simulink model "test_loopback_buf"  (Simulink 6.2)
settings: Solver=ode45  StartTime=0.0  StopTime=4000  RelTol=1e-3
undefined symbols (not defined in the file): Down, Up
libraries: xbsIndex_r3 x1383, xps_library x52, casper_library x37
(part 6 of 8)

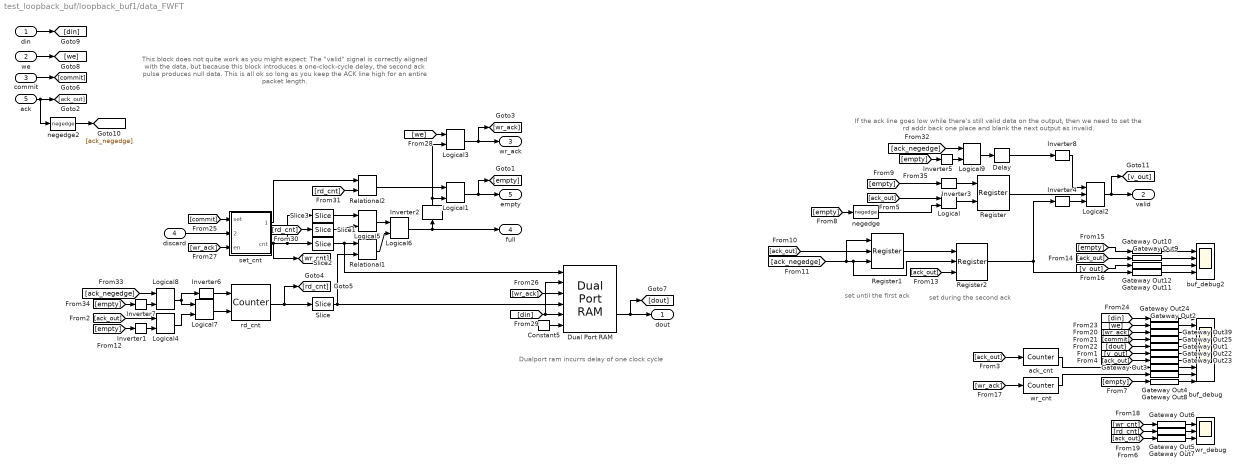
== system test_loopback_buf/loopback_buf1/data_FWFT ==
  note: This block does not quite work as you might expect:
      | The "valid" signal is correctly aligned with the data,
      | but because this block introduces a one-clock-cycle delay,
      | the second ack pulse produces null data.
      |
      | This is all ok so long as you keep the ACK line high for an entire packet length.
  note: set until the first ack
  note: set during the second ack
  note: If the ack line goes low while there's still valid data on the output,
      | then we need to set the rd addr back one place and blank the next
      | output as invalid.
  note: Dualport ram incurrs delay
      | of one clock cycle
  din : Inport  Port=1  LatchInput=off
  we : Inport  Port=2  LatchInput=off
  commit : Inport  Port=3  LatchInput=off
  discard : Inport  Port=4  LatchInput=off
  ack : Inport  Port=5  LatchInput=off
  Constant5 : xbsIndex_r3/Constant  const=0  equ=P=C  arith_type=Boolean  n_bits=1  bin_pt=0  opselect=C  inp2=PCIN>>17  opr=+  inp1=P  carry=CIN  iostate=0  explicit_period=on  period=1  dbl_ovrd=off
  Delay : xbsIndex_r3/Delay  latency=1  reg_retiming=off  explicit_period=off  period=1  en=off  accept_only_valid=off  init_zero=on  dbl_ovrd=off  show_param=off
      settings: xl_area=[0, 0, 0, 0, 0, 0, 0]
  Dual Port RAM : xbsIndex_r3/Dual Port RAM  depth=2^depth_bits  initVector=0  write_mode_A=Read Before Write  write_mode_B=Read Before Write  latency=1  mem_collision=off  init_zero=on  explicit_period=off  period=1  dbl_ovrd=off  rst_a=off  init_a=0  rst_b=off  init_b=0  show_param=off  distributed_mem=off  use_rpm=off  gen_core=off
      settings: xl_area=[0, 0, 0, 0, 0, 0, 0]
  Gateway Out{1..12,22..25,39} (17 alike) : xbsIndex_r3/Gateway Out  output_type=Double  nbits=8  bin_pt=6  arith_type=Boolean  quantization=Truncate  overflow=Wrap  hdl_port=on  timing_constraint=None  locs_specified=off  LOCs={}  needs_fixed_name=off  show_param=off
      settings: xl_area=[0, 0, 0, 0, 0, 0, 0]
  Inverter{1,3..8} (7 alike) : xbsIndex_r3/Inverter  latency=0  explicit_period=off  period=1  en=off  dbl_ovrd=off  show_param=off
      settings: xl_area=[0, 0, 0, 0, 0, 0, 0]
  Inverter2 : xbsIndex_r3/Inverter  Orientation=up  latency=0  explicit_period=off  period=1  en=off  dbl_ovrd=off  show_param=off
      settings: xl_area=[0, 0, 0, 0, 0, 0, 0]
  Logical : xbsIndex_r3/Logical  logical_function=OR  inputs=2  precision=Full  arith_type=Unsigned  n_bits=8  bin_pt=2  align_bp=on  latency=0  explicit_period=off  period=1  en=off  dbl_ovrd=off  show_param=off
      settings: xl_area=[0, 0, 0, 0, 0, 0, 0]
  Logical1 : xbsIndex_r3/Logical  logical_function=AND  inputs=2  precision=Full  arith_type=Unsigned  n_bits=8  bin_pt=2  align_bp=on  latency=0  explicit_period=on  period=1  en=off  dbl_ovrd=off  show_param=off
      settings: xl_area=[0, 0, 0, 0, 0, 0, 0]
  Logical2 : xbsIndex_r3/Logical  logical_function=AND  inputs=3  precision=Full  arith_type=Unsigned  n_bits=8  bin_pt=2  align_bp=on  latency=0  explicit_period=on  period=1  en=off  dbl_ovrd=off  show_param=off
      settings: xl_area=[0, 0, 0, 0, 0, 0, 0]
  Logical{3..4,6,8..9} (5 alike) : xbsIndex_r3/Logical  logical_function=AND  inputs=2  precision=Full  arith_type=Unsigned  n_bits=8  bin_pt=2  align_bp=on  latency=0  explicit_period=off  period=1  en=off  dbl_ovrd=off  show_param=off
      settings: xl_area=[0, 0, 0, 0, 0, 0, 0]
  Logical5 : xbsIndex_r3/Logical  logical_function=XOR  inputs=2  precision=Full  arith_type=Unsigned  n_bits=8  bin_pt=2  align_bp=on  latency=0  explicit_period=off  period=1  en=off  dbl_ovrd=off  show_param=off
      settings: xl_area=[0, 0, 0, 0, 0, 0, 0]
  Logical7 : xbsIndex_r3/Logical  logical_function=OR  inputs=2  precision=Full  arith_type=Unsigned  n_bits=8  bin_pt=2  align_bp=on  latency=0  explicit_period=off  period=1  en=off  dbl_ovrd=off  show_param=off
      settings: xl_area=[0, 0, 0, 0, 0, 0, 0]
  Register : xbsIndex_r3/Register  init=0  reg_only_valid=off  explicit_period=on  period=1  rst=off  en=on  out_en=off  dbl_ovrd=off  show_param=off
      settings: xl_area=[0, 0, 0, 0, 0, 0, 0]
  Register1 : xbsIndex_r3/Register  init=0  reg_only_valid=off  explicit_period=on  period=1  rst=on  en=on  out_en=off  dbl_ovrd=off  show_param=off
      settings: xl_area=[0, 0, 0, 0, 0, 0, 0]
  Register2 : xbsIndex_r3/Register  init=0  reg_only_valid=off  explicit_period=on  period=1  rst=on  en=on  out_en=off  dbl_ovrd=off  show_param=off
      settings: xl_area=[0, 0, 0, 0, 0, 0, 0]
  Relational1 : xbsIndex_r3/Relational  mode=a=b  latency=0  explicit_period=on  period=1  en=off  dbl_ovrd=off  show_param=off
      settings: xl_area=[0, 0, 0, 0, 0, 0, 0]
  Relational2 : xbsIndex_r3/Relational  mode=a=b  latency=0  explicit_period=on  period=1  en=off  dbl_ovrd=off  show_param=off
      settings: xl_area=[0, 0, 0, 0, 0, 0, 0]
  Slice : xbsIndex_r3/Slice  mode=Two Bit Locations  nbits=1  bit1=-1  base1=MSB of Input  bit0=0  base0=LSB of Input  boolean_output=off  explicit_period=off  period=1  dbl_ovrd=off
  Slice1 : xbsIndex_r3/Slice  mode=Upper Bit Location + Width  nbits=1  bit1=0  base1=MSB of Input  bit0=0  base0=LSB of Input  boolean_output=on  explicit_period=off  period=1  dbl_ovrd=off
  Slice2 : xbsIndex_r3/Slice  mode=Two Bit Locations  nbits=1  bit1=-1  base1=MSB of Input  bit0=0  base0=LSB of Input  boolean_output=off  explicit_period=off  period=1  dbl_ovrd=off
  Slice3 : xbsIndex_r3/Slice  mode=Upper Bit Location + Width  nbits=1  bit1=0  base1=MSB of Input  bit0=0  base0=LSB of Input  boolean_output=on  explicit_period=off  period=1  dbl_ovrd=off
  ack_cnt : xbsIndex_r3/Counter  cnt_type=Free Running  n_bits=depth_bits + 1  bin_pt=0  arith_type=Unsigned  start_count=0  cnt_to=Inf  cnt_by_val=1  operation=Up  explicit_period=on  period=1  load_pin=off  rst=off  en=on  dbl_ovrd=off  show_param=off  use_rpm=on  gen_core=off
      settings: xl_area=[0, 0, 0, 0, 0, 0, 0]
  buf_debug : Scope  NumInputPorts=10
      settings: YMin=12000~0~9500~0~15500~-5~-5~-5~-5~-5  YMax=13300~1~10500~1~17250~5~5~5~5~5  SaveName=ScopeData13
  buf_debug2 : Scope  NumInputPorts=4
      settings: YMin=0~1~0~-1  YMax=1~1~1~1  SaveName=ScopeData15
  negedge : casper_library/Misc/negedge  Tag=Rising Edge Detector
  negedge2 : casper_library/Misc/negedge  Tag=Rising Edge Detector
  rd_cnt : xbsIndex_r3/Counter  cnt_type=Free Running  n_bits=depth_bits + 1  bin_pt=0  arith_type=Unsigned  start_count=0  cnt_to=Inf  cnt_by_val=1  operation=Up/Down  explicit_period=on  period=1  load_pin=off  rst=off  en=on  dbl_ovrd=off  show_param=off  use_rpm=on  gen_core=off
      settings: xl_area=[0, 0, 0, 0, 0, 0, 0]
  rd_wr_debug : Scope  NumInputPorts=3
      settings: YMin=12000~0~-5  YMax=13300~1~5  SaveName=ScopeData14
  set_cnt : Subsystem
  wr_cnt : xbsIndex_r3/Counter  cnt_type=Free Running  n_bits=depth_bits + 1  bin_pt=0  arith_type=Unsigned  start_count=0  cnt_to=Inf  cnt_by_val=1  operation=Up  explicit_period=on  period=1  load_pin=off  rst=off  en=on  dbl_ovrd=off  show_param=off  use_rpm=on  gen_core=off
      settings: xl_area=[0, 0, 0, 0, 0, 0, 0]
  dout : Outport
  valid : Outport  Port=2
  wr_ack : Outport  Port=3
  full : Outport  Port=4
  empty : Outport  Port=5
  wires:
  Relational2/1 -> Logical1/1
  Logical6/1 -> Inverter2/1, full/1
  Logical5/1 -> Logical6/1
  Relational1/1 -> Logical6/2
  Slice1/1 -> Logical5/2
  Slice3/1 -> Logical5/1
  Slice2/1 -> Relational1/1, Dual Port RAM/1
  Slice/1 -> Relational1/2, Dual Port RAM/4
  set_cnt/2(cnt) -> Slice3/1, Slice2/1, [wr_cnt]
  set_cnt/1(set_cnt) -> Relational2/1
  rd_cnt/1 -> [rd_cnt], Slice/1
  commit/1 -> [commit]
  Inverter2/1 -> Logical1/2, Logical3/2
  we/1 -> [we]
  discard/1 -> set_cnt/2(undo)
  Constant5/1 -> Dual Port RAM/6
  Dual Port RAM/2 -> dout/1, [dout]
  Logical1/1 -> [empty], empty/1
  Gateway Out24/1 -> buf_debug/1
  Gateway Out2/1 -> buf_debug/2
  Gateway Out39/1 -> buf_debug/3
  Gateway Out25/1 -> buf_debug/4
  Gateway Out1/1 -> buf_debug/5
  Gateway Out22/1 -> buf_debug/6
  Gateway Out23/1 -> buf_debug/7
  Gateway Out3/1 -> buf_debug/8
  Gateway Out4/1 -> buf_debug/9
  ack_cnt/1 -> Gateway Out3/1
  wr_cnt/1 -> Gateway Out4/1
  [empty] -> Inverter1/1
  [v_out] -> Gateway Out22/1
  ack/1 -> [ack_out], negedge2/1
  [ack_out] -> Logical4/1
  [ack_out] -> ack_cnt/1
  [ack_out] -> Gateway Out23/1
  Gateway Out6/1 -> rd_wr_debug/1
  Gateway Out5/1 -> rd_wr_debug/2
  Gateway Out7/1 -> rd_wr_debug/3
  [ack_out] -> Gateway Out7/1
  Gateway Out8/1 -> buf_debug/10
  [empty] -> Gateway Out8/1
  Inverter1/1 -> Logical4/2
  Logical2/1 -> valid/1, [v_out]
  [ack_negedge] -> Register1/1, Register1/3, Register2/2
  [ack_out] -> Register1/2
  Register1/1 -> Register2/1
  Gateway Out10/1 -> buf_debug2/1
  Gateway Out9/1 -> buf_debug2/2
  Gateway Out12/1 -> buf_debug2/3
  Gateway Out11/1 -> buf_debug2/4
  [ack_out] -> Gateway Out9/1
  [empty] -> Gateway Out10/1
  [v_out] -> Gateway Out12/1
  [ack_out] -> Register2/3
  [wr_ack] -> wr_cnt/1
  [wr_cnt] -> Gateway Out6/1
  [rd_cnt] -> Gateway Out5/1
  [wr_ack] -> Gateway Out39/1
  [commit] -> Gateway Out25/1
  [dout] -> Gateway Out1/1
  [we] -> Gateway Out2/1
  [din] -> Gateway Out24/1
  [commit] -> set_cnt/1(set)
  [wr_ack] -> Dual Port RAM/3
  [wr_ack] -> set_cnt/3(en)
  [we] -> Logical3/1
  Logical3/1 -> wr_ack/1, [wr_ack]
  [din] -> Dual Port RAM/2, Dual Port RAM/5
  din/1 -> [din]
  [rd_cnt] -> Slice1/1
  [rd_cnt] -> Relational2/2
  Register2/1 -> Gateway Out11/1, Inverter4/1
  negedge2/1 -> [ack_negedge]
  Inverter6/1 -> rd_cnt/1
  Logical7/1 -> rd_cnt/2
  Logical4/1 -> Logical7/2
  Logical8/1 -> Inverter6/1, Logical7/1
  [ack_negedge] -> Logical8/1
  [empty] -> Inverter7/1
  Inverter7/1 -> Logical8/2
  [ack_negedge] -> Logical9/1
  [empty] -> Inverter5/1
  Inverter5/1 -> Logical9/2
  Logical9/1 -> Delay/1
  Delay/1 -> Inverter8/1
  Inverter3/1 -> Register/1
  [empty] -> Inverter3/1
  Logical/1 -> Register/2
  [empty] -> negedge/1
  [ack_out] -> Logical/1
  negedge/1 -> Logical/2
  Inverter4/1 -> Logical2/3
  Inverter8/1 -> Logical2/1
  Register/1 -> Logical2/2

== system test_loopback_buf/loopback_mux0/Subsystem15 ==
  rst : Inport  Port=1  LatchInput=off
  we : Inport  Port=2  LatchInput=off
  eof : Inport  Port=3  LatchInput=off
  Constant : xbsIndex_r3/Constant  const=payload_len -1  equ=P=C  arith_type=Unsigned  n_bits=8  bin_pt=0  opselect=C  inp2=PCIN>>17  opr=+  inp1=P  carry=CIN  iostate=0  explicit_period=off  period=1  dbl_ovrd=off
  Delay1 : xbsIndex_r3/Delay  latency=1  reg_retiming=on  explicit_period=off  period=1  en=off  accept_only_valid=off  init_zero=on  dbl_ovrd=off  show_param=off
      settings: xl_area=[0, 0, 0, 0, 0, 0, 0]
  Delay15 : xbsIndex_r3/Delay  latency=1  reg_retiming=on  explicit_period=off  period=1  en=off  accept_only_valid=off  init_zero=on  dbl_ovrd=off  show_param=off
      settings: xl_area=[0, 0, 0, 0, 0, 0, 0]
  Delay2 : xbsIndex_r3/Delay  latency=1  reg_retiming=on  explicit_period=off  period=1  en=off  accept_only_valid=off  init_zero=on  dbl_ovrd=off  show_param=off
      settings: xl_area=[0, 0, 0, 0, 0, 0, 0]
  Gateway Out{23..27} (5 alike) : xbsIndex_r3/Gateway Out  output_type=Double  nbits=8  bin_pt=6  arith_type=Boolean  quantization=Truncate  overflow=Wrap  hdl_port=on  timing_constraint=None  locs_specified=off  LOCs={}  needs_fixed_name=off  show_param=off
      settings: xl_area=[0, 0, 0, 0, 0, 0, 0]
  Logical1 : xbsIndex_r3/Logical  logical_function=AND  inputs=2  precision=Full  arith_type=Unsigned  n_bits=8  bin_pt=2  align_bp=on  latency=0  explicit_period=on  period=1  en=off  dbl_ovrd=off  show_param=off
      settings: xl_area=[0, 0, 0, 0, 0, 0, 0]
  Logical2 : xbsIndex_r3/Logical  logical_function=AND  inputs=2  precision=Full  arith_type=Unsigned  n_bits=8  bin_pt=2  align_bp=on  latency=0  explicit_period=on  period=1  en=off  dbl_ovrd=off  show_param=off
      settings: xl_area=[0, 0, 0, 0, 0, 0, 0]
  Relational : xbsIndex_r3/Relational  mode=a!=b  latency=0  explicit_period=off  period=1  en=off  dbl_ovrd=off  show_param=off
      settings: xl_area=[0, 0, 0, 0, 0, 0, 0]
  Scope2 : Scope  NumInputPorts=5
      settings: TimeRange=10000  YMin=0~0~0~0~-1  YMax=5000~1~3~1~1  SaveName=ScopeData2
  payload_cnt1 : xbsIndex_r3/Counter  cnt_type=Free Running  n_bits=32  bin_pt=0  arith_type=Unsigned  start_count=0  cnt_to=0  cnt_by_val=1  operation=Up  explicit_period=on  period=1  load_pin=off  rst=on  en=on  dbl_ovrd=off  show_param=off  use_rpm=on  gen_core=off
      settings: xl_area=[0, 0, 0, 0, 0, 0, 0]
  payload_cnt2 : xbsIndex_r3/Counter  cnt_type=Free Running  n_bits=8  bin_pt=0  arith_type=Unsigned  start_count=0  cnt_to=0  cnt_by_val=1  operation=Up  explicit_period=on  period=1  load_pin=off  rst=on  en=on  dbl_ovrd=off  show_param=off  use_rpm=on  gen_core=off
      settings: xl_area=[0, 0, 0, 0, 0, 0, 0]
  err_cnt : Outport
  err : Outport  Port=2
  wires:
  payload_cnt1/1 -> err_cnt/1, Gateway Out27/1
  rst/1 -> Delay15/1
  [rst] -> payload_cnt1/1
  we/1 -> Delay1/1
  eof/1 -> Delay2/1
  Logical2/1 -> payload_cnt2/1, Logical1/1
  payload_cnt2/1 -> Relational/2, Gateway Out25/1
  [we] -> Logical2/1, payload_cnt2/2
  [eof] -> Logical2/2
  Constant/1 -> Relational/1
  Relational/1 -> Logical1/2, Gateway Out26/1
  Logical1/1 -> payload_cnt1/2, err/1
  Gateway Out23/1 -> Scope2/1
  Gateway Out24/1 -> Scope2/2
  Gateway Out25/1 -> Scope2/3
  Gateway Out26/1 -> Scope2/4
  Gateway Out27/1 -> Scope2/5
  [we] -> Gateway Out23/1
  [eof] -> Gateway Out24/1
  Delay15/1 -> [rst]
  Delay1/1 -> [we]
  Delay2/1 -> [eof]

== system test_loopback_buf/loopback_mux0/snap ==
  note: could not route with
      | brams size2^14
  data_in : Inport  Port=1  LatchInput=off
  we : Inport  Port=2  LatchInput=off
  trig : Inport  Port=3  LatchInput=off
  Constant1 : xbsIndex_r3/Constant  const=1  equ=P=C  arith_type=Boolean  n_bits=1  bin_pt=0  opselect=C  inp2=PCIN>>17  opr=+  inp1=P  carry=CIN  iostate=0  explicit_period=on  period=1  dbl_ovrd=off
  Constant2 : xbsIndex_r3/Constant  const=1  equ=P=C  arith_type=Boolean  n_bits=1  bin_pt=0  opselect=C  inp2=PCIN>>17  opr=+  inp1=P  carry=CIN  iostate=0  explicit_period=on  period=1  dbl_ovrd=off
  Constant3 : Constant  Value=0
  Counter : xbsIndex_r3/Counter  cnt_type=Free Running  n_bits=32  bin_pt=0  arith_type=Unsigned  start_count=1  cnt_to=Inf  cnt_by_val=1  operation=Up  explicit_period=on  period=1  load_pin=off  rst=on  en=on  dbl_ovrd=off  show_param=off  use_rpm=on  gen_core=off
      settings: xl_area=[0, 0, 0, 0, 0, 0, 0]
  Delay2 : xbsIndex_r3/Delay  latency=2  reg_retiming=on  explicit_period=on  period=1  en=off  accept_only_valid=off  init_zero=on  dbl_ovrd=off  show_param=off
      settings: xl_area=[0, 0, 0, 0, 0, 0, 0]
  Delay{3..7} (5 alike) : xbsIndex_r3/Delay  latency=1  reg_retiming=on  explicit_period=on  period=1  en=off  accept_only_valid=off  init_zero=on  dbl_ovrd=off  show_param=off
      settings: xl_area=[0, 0, 0, 0, 0, 0, 0]
  Gateway Out{1,5..10} (7 alike) : xbsIndex_r3/Gateway Out  output_type=Double  nbits=8  bin_pt=6  arith_type=Boolean  quantization=Truncate  overflow=Wrap  hdl_port=off  timing_constraint=None  locs_specified=off  LOCs={}  needs_fixed_name=off  show_param=off
      settings: xl_area=[0, 0, 0, 0, 0, 0, 0]
  Inverter : xbsIndex_r3/Inverter  latency=0  explicit_period=off  period=1  en=off  dbl_ovrd=off  show_param=off
      settings: xl_area=[0, 0, 0, 0, 0, 0, 0]
  Logical1 : xbsIndex_r3/Logical  logical_function=AND  inputs=2  precision=Full  arith_type=Unsigned  n_bits=8  bin_pt=2  align_bp=on  latency=0  explicit_period=off  period=1  en=off  dbl_ovrd=off  show_param=off
      settings: xl_area=[0, 0, 0, 0, 0, 0, 0]
  Logical2 : xbsIndex_r3/Logical  logical_function=OR  inputs=2  precision=Full  arith_type=Unsigned  n_bits=8  bin_pt=2  align_bp=on  latency=0  explicit_period=on  period=1  en=off  dbl_ovrd=off  show_param=off
      settings: xl_area=[0, 0, 0, 0, 0, 0, 0]
  Logical3 : xbsIndex_r3/Logical  logical_function=OR  inputs=3  precision=Full  arith_type=Unsigned  n_bits=8  bin_pt=2  align_bp=on  latency=0  explicit_period=on  period=1  en=off  dbl_ovrd=off  show_param=off
      settings: xl_area=[0, 0, 0, 0, 0, 0, 0]
  Logical4 : xbsIndex_r3/Logical  logical_function=AND  inputs=2  precision=Full  arith_type=Unsigned  n_bits=8  bin_pt=2  align_bp=on  latency=0  explicit_period=on  period=1  en=off  dbl_ovrd=off  show_param=off
      settings: xl_area=[0, 0, 0, 0, 0, 0, 0]
  Mux1 : xbsIndex_r3/Mux  inputs=2  precision=Full  arith_type="Signed  (2's comp)"  n_bits=8  bin_pt=2  quantization=Truncate  overflow=Wrap  latency=0  explicit_period=off  period=1  en=off  dbl_ovrd=off  show_param=off  mux_type=off  use_rpm=off  gen_core=off
      settings: xl_area=[0, 0, 0, 0, 0, 0, 0]
  Mux2 : xbsIndex_r3/Mux  inputs=2  precision=Full  arith_type="Signed  (2's comp)"  n_bits=8  bin_pt=2  quantization=Truncate  overflow=Wrap  latency=0  explicit_period=off  period=1  en=off  dbl_ovrd=off  show_param=off  mux_type=off  use_rpm=off  gen_core=off
      settings: xl_area=[0, 0, 0, 0, 0, 0, 0]
  Pulse Generator1 : DiscretePulseGenerator  Period=4196  PulseWidth=2
  Register : xbsIndex_r3/Register  init=0  reg_only_valid=off  explicit_period=off  period=1  rst=on  en=on  out_en=off  dbl_ovrd=off  show_param=off
      settings: xl_area=[0, 0, 0, 0, 0, 0, 0]
  Register1 : xbsIndex_r3/Register  init=0  reg_only_valid=off  explicit_period=off  period=1  rst=on  en=on  out_en=off  dbl_ovrd=off  show_param=off
      settings: xl_area=[0, 0, 0, 0, 0, 0, 0]
  Register2 : xbsIndex_r3/Register  init=0  reg_only_valid=off  explicit_period=off  period=1  rst=on  en=on  out_en=off  dbl_ovrd=off  show_param=off
      settings: xl_area=[0, 0, 0, 0, 0, 0, 0]
  Reinterpret : xbsIndex_r3/Reinterpret  force_arith_type=on  arith_type=Unsigned  force_bin_pt=on  bin_pt=0  force_valid=on
  Relational : xbsIndex_r3/Relational  mode=a>=b  latency=0  explicit_period=on  period=1  en=off  dbl_ovrd=off  show_param=off
      settings: xl_area=[0, 0, 0, 0, 0, 0, 0]
  Scope2 : Scope  NumInputPorts=7
      settings: YMin=2.72014e+008~0~0~-5~-5~-5~-5  YMax=3.00648e+008~110~1~5~5~5~5  SaveName=ScopeData3
  addr : xps_library/software register  Tag=xps:sw_reg  io_dir=To Processor  arith_type=Unsigned  bitwidth=32  bin_pt=0  sample_period=1  gw_name=b_2x_8a_r310_a_loopback_mux0_snap_addr_user_data_in
  bram : xps_library/Shared BRAM  Tag=xps:bram  arith_type=Unsigned  addr_width=nsamples  data_width=32  data_bin_pt=0  init_vals=0  sample_rate=1
  ctrl : xps_library/software register  Tag=xps:sw_reg  io_dir=From Processor  arith_type=Unsigned  bitwidth=32  bin_pt=0  sample_period=1  gw_name=b_2x_8a_r310_a_loopback_mux0_snap_ctrl_user_data_out
  enable : xbsIndex_r3/Slice  mode=Lower Bit Location + Width  nbits=1  bit1=0  base1=LSB of Input  bit0=0  base0=LSB of Input  boolean_output=on  explicit_period=on  period=1  dbl_ovrd=off
  freeze_cntr : casper_library/Misc/freeze_cntr  CounterBits=nsamples
  posedge : casper_library/Misc/posedge  Tag=Rising Edge Detector
  trig1 : xbsIndex_r3/Slice  mode=Lower Bit Location + Width  nbits=1  bit1=0  base1=LSB of Input  bit0=1  base0=LSB of Input  boolean_output=on  explicit_period=off  period=1  dbl_ovrd=off
  trig_offset : xps_library/software register  Tag=xps:sw_reg  io_dir=From Processor  arith_type=Unsigned  bitwidth=32  bin_pt=0  sample_period=1  gw_name=b_2x_8a_r310_a_loopback_mux0_snap_trig_offset_user_data_out
  valid : xbsIndex_r3/Slice  mode=Lower Bit Location + Width  nbits=1  bit1=0  base1=LSB of Input  bit0=2  base0=LSB of Input  boolean_output=on  explicit_period=off  period=1  dbl_ovrd=off
  wires:
  data_in/1 -> Reinterpret/1
  freeze_cntr/1 -> Register1/1, bram/1
  Register/1 -> Gateway Out7/1, freeze_cntr/2
  Mux2/1 -> Logical1/1, Gateway Out10/1
  Inverter/1 -> Logical1/2
  valid/1 -> Mux1/1
  trig1/1 -> Mux2/1
  Register1/1 -> addr/1
  Constant2/1 -> Mux1/3
  we/1 -> Mux1/2
  Mux1/1 -> Delay5/1, Counter/2
  Constant1/1 -> Mux2/3
  posedge/1 -> Inverter/1, Register2/2, Delay4/1, Register1/2, Logical3/3, Delay2/1
  ctrl/1 -> trig1/1, valid/1, enable/1
  freeze_cntr/2 -> Register1/3, bram/3, Gateway Out1/1
  enable/1 -> posedge/1
  trig/1 -> Mux2/2
  Logical4/1 -> Register/2, Gateway Out8/1
  Logical1/1 -> Register2/1, Logical2/1, Counter/1, Gateway Out5/1, Register2/3
  Delay3/1 -> bram/2
  Register2/1 -> Logical2/2
  Delay4/1 -> Logical3/1
  Logical3/1 -> Register/3, Register/1, Gateway Out6/1
  Constant3/1 -> trig_offset/1
  trig_offset/1 -> Relational/2
  Relational/1 -> Logical4/2
  Logical2/1 -> Gateway Out9/1, Delay6/1
  Counter/1 -> Delay7/1
  Delay2/1 -> Logical3/2
  Delay5/1 -> freeze_cntr/1
  Delay6/1 -> Logical4/1
  Delay7/1 -> Relational/1
  Gateway Out9/1 -> Scope2/3
  Gateway Out5/1 -> Scope2/2
  Gateway Out8/1 -> Scope2/4
  Gateway Out6/1 -> Scope2/5
  Gateway Out10/1 -> Scope2/1
  Gateway Out7/1 -> Scope2/6
  Pulse Generator1/1 -> ctrl/1
  Gateway Out1/1 -> Scope2/7
  Reinterpret/1 -> Delay3/1

== system test_loopback_buf/loopback_poor_timing/Subsystem15 ==
  rst : Inport  Port=1  LatchInput=off
  we : Inport  Port=2  LatchInput=off
  eof : Inport  Port=3  LatchInput=off
  Constant : xbsIndex_r3/Constant  const=payload_len -1  equ=P=C  arith_type=Unsigned  n_bits=8  bin_pt=0  opselect=C  inp2=PCIN>>17  opr=+  inp1=P  carry=CIN  iostate=0  explicit_period=off  period=1  dbl_ovrd=off
  Delay1 : xbsIndex_r3/Delay  latency=1  reg_retiming=on  explicit_period=off  period=1  en=off  accept_only_valid=off  init_zero=on  dbl_ovrd=off  show_param=off
      settings: xl_area=[0, 0, 0, 0, 0, 0, 0]
  Delay15 : xbsIndex_r3/Delay  latency=1  reg_retiming=on  explicit_period=off  period=1  en=off  accept_only_valid=off  init_zero=on  dbl_ovrd=off  show_param=off
      settings: xl_area=[0, 0, 0, 0, 0, 0, 0]
  Delay2 : xbsIndex_r3/Delay  latency=1  reg_retiming=on  explicit_period=off  period=1  en=off  accept_only_valid=off  init_zero=on  dbl_ovrd=off  show_param=off
      settings: xl_area=[0, 0, 0, 0, 0, 0, 0]
  Gateway Out{23..27} (5 alike) : xbsIndex_r3/Gateway Out  output_type=Double  nbits=8  bin_pt=6  arith_type=Boolean  quantization=Truncate  overflow=Wrap  hdl_port=on  timing_constraint=None  locs_specified=off  LOCs={}  needs_fixed_name=off  show_param=off
      settings: xl_area=[0, 0, 0, 0, 0, 0, 0]
  Logical1 : xbsIndex_r3/Logical  logical_function=AND  inputs=2  precision=Full  arith_type=Unsigned  n_bits=8  bin_pt=2  align_bp=on  latency=0  explicit_period=on  period=1  en=off  dbl_ovrd=off  show_param=off
      settings: xl_area=[0, 0, 0, 0, 0, 0, 0]
  Logical2 : xbsIndex_r3/Logical  logical_function=AND  inputs=2  precision=Full  arith_type=Unsigned  n_bits=8  bin_pt=2  align_bp=on  latency=0  explicit_period=on  period=1  en=off  dbl_ovrd=off  show_param=off
      settings: xl_area=[0, 0, 0, 0, 0, 0, 0]
  Relational : xbsIndex_r3/Relational  mode=a!=b  latency=0  explicit_period=off  period=1  en=off  dbl_ovrd=off  show_param=off
      settings: xl_area=[0, 0, 0, 0, 0, 0, 0]
  Scope2 : Scope  NumInputPorts=5
      settings: TimeRange=10000  YMin=0~0~0~0~-1  YMax=5000~1~3~1~1  SaveName=ScopeData2
  payload_cnt1 : xbsIndex_r3/Counter  cnt_type=Free Running  n_bits=32  bin_pt=0  arith_type=Unsigned  start_count=0  cnt_to=0  cnt_by_val=1  operation=Up  explicit_period=on  period=1  load_pin=off  rst=on  en=on  dbl_ovrd=off  show_param=off  use_rpm=on  gen_core=off
      settings: xl_area=[0, 0, 0, 0, 0, 0, 0]
  payload_cnt2 : xbsIndex_r3/Counter  cnt_type=Free Running  n_bits=8  bin_pt=0  arith_type=Unsigned  start_count=0  cnt_to=0  cnt_by_val=1  operation=Up  explicit_period=on  period=1  load_pin=off  rst=on  en=on  dbl_ovrd=off  show_param=off  use_rpm=on  gen_core=off
      settings: xl_area=[0, 0, 0, 0, 0, 0, 0]
  err_cnt : Outport
  err : Outport  Port=2
  wires:
  payload_cnt1/1 -> err_cnt/1, Gateway Out27/1
  rst/1 -> Delay15/1
  [rst] -> payload_cnt1/1
  we/1 -> Delay1/1
  eof/1 -> Delay2/1
  Logical2/1 -> payload_cnt2/1, Logical1/1
  payload_cnt2/1 -> Relational/2, Gateway Out25/1
  [we] -> Logical2/1, payload_cnt2/2
  [eof] -> Logical2/2
  Constant/1 -> Relational/1
  Relational/1 -> Logical1/2, Gateway Out26/1
  Logical1/1 -> payload_cnt1/2, err/1
  Gateway Out23/1 -> Scope2/1
  Gateway Out24/1 -> Scope2/2
  Gateway Out25/1 -> Scope2/3
  Gateway Out26/1 -> Scope2/4
  Gateway Out27/1 -> Scope2/5
  [we] -> Gateway Out23/1
  [eof] -> Gateway Out24/1
  Delay15/1 -> [rst]
  Delay1/1 -> [we]
  Delay2/1 -> [eof]

== system test_loopback_buf/loopback_poor_timing/snap ==
  note: could not route with
      | brams size2^14
  data_in : Inport  Port=1  LatchInput=off
  we : Inport  Port=2  LatchInput=off
  trig : Inport  Port=3  LatchInput=off
  Constant1 : xbsIndex_r3/Constant  const=1  equ=P=C  arith_type=Boolean  n_bits=1  bin_pt=0  opselect=C  inp2=PCIN>>17  opr=+  inp1=P  carry=CIN  iostate=0  explicit_period=on  period=1  dbl_ovrd=off
  Constant2 : xbsIndex_r3/Constant  const=1  equ=P=C  arith_type=Boolean  n_bits=1  bin_pt=0  opselect=C  inp2=PCIN>>17  opr=+  inp1=P  carry=CIN  iostate=0  explicit_period=on  period=1  dbl_ovrd=off
  Constant3 : Constant  Value=0
  Counter : xbsIndex_r3/Counter  cnt_type=Free Running  n_bits=32  bin_pt=0  arith_type=Unsigned  start_count=1  cnt_to=Inf  cnt_by_val=1  operation=Up  explicit_period=on  period=1  load_pin=off  rst=on  en=on  dbl_ovrd=off  show_param=off  use_rpm=on  gen_core=off
      settings: xl_area=[0, 0, 0, 0, 0, 0, 0]
  Delay2 : xbsIndex_r3/Delay  latency=2  reg_retiming=on  explicit_period=on  period=1  en=off  accept_only_valid=off  init_zero=on  dbl_ovrd=off  show_param=off
      settings: xl_area=[0, 0, 0, 0, 0, 0, 0]
  Delay{3..7} (5 alike) : xbsIndex_r3/Delay  latency=1  reg_retiming=on  explicit_period=on  period=1  en=off  accept_only_valid=off  init_zero=on  dbl_ovrd=off  show_param=off
      settings: xl_area=[0, 0, 0, 0, 0, 0, 0]
  Gateway Out{1,5..10} (7 alike) : xbsIndex_r3/Gateway Out  output_type=Double  nbits=8  bin_pt=6  arith_type=Boolean  quantization=Truncate  overflow=Wrap  hdl_port=off  timing_constraint=None  locs_specified=off  LOCs={}  needs_fixed_name=off  show_param=off
      settings: xl_area=[0, 0, 0, 0, 0, 0, 0]
  Inverter : xbsIndex_r3/Inverter  latency=0  explicit_period=off  period=1  en=off  dbl_ovrd=off  show_param=off
      settings: xl_area=[0, 0, 0, 0, 0, 0, 0]
  Logical1 : xbsIndex_r3/Logical  logical_function=AND  inputs=2  precision=Full  arith_type=Unsigned  n_bits=8  bin_pt=2  align_bp=on  latency=0  explicit_period=off  period=1  en=off  dbl_ovrd=off  show_param=off
      settings: xl_area=[0, 0, 0, 0, 0, 0, 0]
  Logical2 : xbsIndex_r3/Logical  logical_function=OR  inputs=2  precision=Full  arith_type=Unsigned  n_bits=8  bin_pt=2  align_bp=on  latency=0  explicit_period=on  period=1  en=off  dbl_ovrd=off  show_param=off
      settings: xl_area=[0, 0, 0, 0, 0, 0, 0]
  Logical3 : xbsIndex_r3/Logical  logical_function=OR  inputs=3  precision=Full  arith_type=Unsigned  n_bits=8  bin_pt=2  align_bp=on  latency=0  explicit_period=on  period=1  en=off  dbl_ovrd=off  show_param=off
      settings: xl_area=[0, 0, 0, 0, 0, 0, 0]
  Logical4 : xbsIndex_r3/Logical  logical_function=AND  inputs=2  precision=Full  arith_type=Unsigned  n_bits=8  bin_pt=2  align_bp=on  latency=0  explicit_period=on  period=1  en=off  dbl_ovrd=off  show_param=off
      settings: xl_area=[0, 0, 0, 0, 0, 0, 0]
  Mux1 : xbsIndex_r3/Mux  inputs=2  precision=Full  arith_type="Signed  (2's comp)"  n_bits=8  bin_pt=2  quantization=Truncate  overflow=Wrap  latency=0  explicit_period=off  period=1  en=off  dbl_ovrd=off  show_param=off  mux_type=off  use_rpm=off  gen_core=off
      settings: xl_area=[0, 0, 0, 0, 0, 0, 0]
  Mux2 : xbsIndex_r3/Mux  inputs=2  precision=Full  arith_type="Signed  (2's comp)"  n_bits=8  bin_pt=2  quantization=Truncate  overflow=Wrap  latency=0  explicit_period=off  period=1  en=off  dbl_ovrd=off  show_param=off  mux_type=off  use_rpm=off  gen_core=off
      settings: xl_area=[0, 0, 0, 0, 0, 0, 0]
  Pulse Generator1 : DiscretePulseGenerator  Period=4196  PulseWidth=2
  Register : xbsIndex_r3/Register  init=0  reg_only_valid=off  explicit_period=off  period=1  rst=on  en=on  out_en=off  dbl_ovrd=off  show_param=off
      settings: xl_area=[0, 0, 0, 0, 0, 0, 0]
  Register1 : xbsIndex_r3/Register  init=0  reg_only_valid=off  explicit_period=off  period=1  rst=on  en=on  out_en=off  dbl_ovrd=off  show_param=off
      settings: xl_area=[0, 0, 0, 0, 0, 0, 0]
  Register2 : xbsIndex_r3/Register  init=0  reg_only_valid=off  explicit_period=off  period=1  rst=on  en=on  out_en=off  dbl_ovrd=off  show_param=off
      settings: xl_area=[0, 0, 0, 0, 0, 0, 0]
  Reinterpret : xbsIndex_r3/Reinterpret  force_arith_type=on  arith_type=Unsigned  force_bin_pt=on  bin_pt=0  force_valid=on
  Relational : xbsIndex_r3/Relational  mode=a>=b  latency=0  explicit_period=on  period=1  en=off  dbl_ovrd=off  show_param=off
      settings: xl_area=[0, 0, 0, 0, 0, 0, 0]
  Scope2 : Scope  NumInputPorts=7
      settings: YMin=2.72014e+008~0~0~-5~-5~-5~-5  YMax=3.00648e+008~110~1~5~5~5~5  SaveName=ScopeData3
  addr : xps_library/software register  Tag=xps:sw_reg  io_dir=To Processor  arith_type=Unsigned  bitwidth=32  bin_pt=0  sample_period=1  gw_name=test_loopback_buf_loopback_poor_timing_snap_addr_user_data_in
  bram : xps_library/Shared BRAM  Tag=xps:bram  arith_type=Unsigned  addr_width=nsamples  data_width=32  data_bin_pt=0  init_vals=0  sample_rate=1
  ctrl : xps_library/software register  Tag=xps:sw_reg  io_dir=From Processor  arith_type=Unsigned  bitwidth=32  bin_pt=0  sample_period=1  gw_name=test_loopback_buf_loopback_poor_timing_snap_ctrl_user_data_out
  enable : xbsIndex_r3/Slice  mode=Lower Bit Location + Width  nbits=1  bit1=0  base1=LSB of Input  bit0=0  base0=LSB of Input  boolean_output=on  explicit_period=on  period=1  dbl_ovrd=off
  freeze_cntr : casper_library/Misc/freeze_cntr  CounterBits=nsamples
  posedge : casper_library/Misc/posedge  Tag=Rising Edge Detector
  trig1 : xbsIndex_r3/Slice  mode=Lower Bit Location + Width  nbits=1  bit1=0  base1=LSB of Input  bit0=1  base0=LSB of Input  boolean_output=on  explicit_period=off  period=1  dbl_ovrd=off
  trig_offset : xps_library/software register  Tag=xps:sw_reg  io_dir=From Processor  arith_type=Unsigned  bitwidth=32  bin_pt=0  sample_period=1  gw_name=test_loopback_buf_loopback_poor_timing_snap_trig_offset_user_data_out
  valid : xbsIndex_r3/Slice  mode=Lower Bit Location + Width  nbits=1  bit1=0  base1=LSB of Input  bit0=2  base0=LSB of Input  boolean_output=on  explicit_period=off  period=1  dbl_ovrd=off
  wires:
  data_in/1 -> Reinterpret/1
  freeze_cntr/1 -> Register1/1, bram/1
  Register/1 -> Gateway Out7/1, freeze_cntr/2
  Mux2/1 -> Logical1/1, Gateway Out10/1
  Inverter/1 -> Logical1/2
  valid/1 -> Mux1/1
  trig1/1 -> Mux2/1
  Register1/1 -> addr/1
  Constant2/1 -> Mux1/3
  we/1 -> Mux1/2
  Mux1/1 -> Delay5/1, Counter/2
  Constant1/1 -> Mux2/3
  posedge/1 -> Inverter/1, Register2/2, Delay4/1, Register1/2, Logical3/3, Delay2/1
  ctrl/1 -> trig1/1, valid/1, enable/1
  freeze_cntr/2 -> Register1/3, bram/3, Gateway Out1/1
  enable/1 -> posedge/1
  trig/1 -> Mux2/2
  Logical4/1 -> Register/2, Gateway Out8/1
  Logical1/1 -> Register2/1, Logical2/1, Counter/1, Gateway Out5/1, Register2/3
  Delay3/1 -> bram/2
  Register2/1 -> Logical2/2
  Delay4/1 -> Logical3/1
  Logical3/1 -> Register/3, Register/1, Gateway Out6/1
  Constant3/1 -> trig_offset/1
  trig_offset/1 -> Relational/2
  Relational/1 -> Logical4/2
  Logical2/1 -> Gateway Out9/1, Delay6/1
  Counter/1 -> Delay7/1
  Delay2/1 -> Logical3/2
  Delay5/1 -> freeze_cntr/1
  Delay6/1 -> Logical4/1
  Delay7/1 -> Relational/1
  Gateway Out9/1 -> Scope2/3
  Gateway Out5/1 -> Scope2/2
  Gateway Out8/1 -> Scope2/4
  Gateway Out6/1 -> Scope2/5
  Gateway Out10/1 -> Scope2/1
  Gateway Out7/1 -> Scope2/6
  Pulse Generator1/1 -> ctrl/1
  Gateway Out1/1 -> Scope2/7
  Reinterpret/1 -> Delay3/1

== system test_loopback_buf/mux_pkts_orig/state_mach ==
  note: state
  note: output
  gbe_valid : Inport  Port=1  LatchInput=off
  pkt_rdy : Inport  Port=2  LatchInput=off
  eof : Inport  Port=3  LatchInput=off
  Constant4 : xbsIndex_r3/Constant  const=1  equ=P=C  arith_type=Boolean  n_bits=1  bin_pt=0  opselect=C  inp2=PCIN>>17  opr=+  inp1=P  carry=CIN  iostate=0  explicit_period=on  period=1  dbl_ovrd=off
  Convert : xbsIndex_r3/Convert  arith_type=Boolean  n_bits=8  bin_pt=6  quantization=Truncate  overflow=Wrap  latency=0  explicit_period=off  period=1  dbl_ovrd=off  show_param=off  inserted_by_tool=off  pipeline=off
      settings: xl_area=[0, 0, 0, 0, 0, 0, 0]
  Inverter : xbsIndex_r3/Inverter  latency=0  explicit_period=off  period=1  en=off  dbl_ovrd=off  show_param=off
      settings: xl_area=[0, 0, 0, 0, 0, 0, 0]
  Inverter1 : xbsIndex_r3/Inverter  Orientation=left  latency=0  explicit_period=off  period=1  en=off  dbl_ovrd=off  show_param=off
      settings: xl_area=[0, 0, 0, 0, 0, 0, 0]
  Inverter2 : xbsIndex_r3/Inverter  latency=0  explicit_period=off  period=1  en=off  dbl_ovrd=off  show_param=off
      settings: xl_area=[0, 0, 0, 0, 0, 0, 0]
  Logical1 : xbsIndex_r3/Logical  logical_function=AND  inputs=2  precision=Full  arith_type=Unsigned  n_bits=8  bin_pt=2  align_bp=on  latency=0  explicit_period=off  period=1  en=off  dbl_ovrd=off  show_param=off
      settings: xl_area=[0, 0, 0, 0, 0, 0, 0]
  Logical2 : xbsIndex_r3/Logical  logical_function=OR  inputs=2  precision=Full  arith_type=Unsigned  n_bits=8  bin_pt=2  align_bp=on  latency=0  explicit_period=off  period=1  en=off  dbl_ovrd=off  show_param=off
      settings: xl_area=[0, 0, 0, 0, 0, 0, 0]
  Logical3 : xbsIndex_r3/Logical  logical_function=AND  inputs=2  precision=Full  arith_type=Unsigned  n_bits=8  bin_pt=2  align_bp=on  latency=0  explicit_period=off  period=1  en=off  dbl_ovrd=off  show_param=off
      settings: xl_area=[0, 0, 0, 0, 0, 0, 0]
  Logical4 : xbsIndex_r3/Logical  logical_function=AND  inputs=2  precision=Full  arith_type=Unsigned  n_bits=8  bin_pt=2  align_bp=on  latency=0  explicit_period=off  period=1  en=off  dbl_ovrd=off  show_param=off
      settings: xl_area=[0, 0, 0, 0, 0, 0, 0]
  Register1 : xbsIndex_r3/Register  init=0  reg_only_valid=off  explicit_period=on  period=1  rst=on  en=on  out_en=off  dbl_ovrd=off  show_param=off
      settings: xl_area=[0, 0, 0, 0, 0, 0, 0]
  Register2 : xbsIndex_r3/Register  init=0  reg_only_valid=off  explicit_period=on  period=1  rst=off  en=on  out_en=off  dbl_ovrd=off  show_param=off
      settings: xl_area=[0, 0, 0, 0, 0, 0, 0]
  gbe_ack : Outport
  loop_ack : Outport  Port=2
  state : Outport  Port=3
  wires:
  Register1/1 -> Convert/1
  Constant4/1 -> Register1/1
  Logical2/1 -> Logical3/2, Register1/3
  Logical3/1 -> Register2/2
  Inverter2/1 -> Register2/1
  gbe_valid/1 -> Logical2/1
  Register2/1 -> Inverter/1, Logical4/2
  Inverter1/1 -> Logical3/1
  eof/1 -> Register1/2
  Inverter/1 -> Logical1/2
  Logical1/1 -> loop_ack/1
  Logical4/1 -> gbe_ack/1
  pkt_rdy/1 -> Logical2/2, Inverter2/1
  Convert/1 -> state/1, Logical1/1, Logical4/1, Inverter1/1

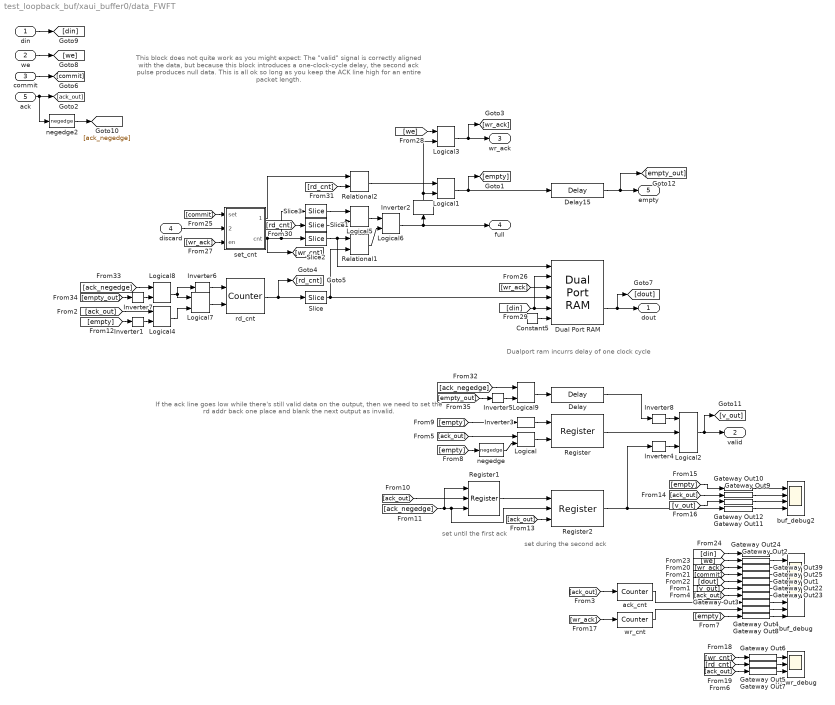
== system test_loopback_buf/xaui_buffer0/data_FWFT ==
  note: This block does not quite work as you might expect:
      | The "valid" signal is correctly aligned with the data,
      | but because this block introduces a one-clock-cycle delay,
      | the second ack pulse produces null data.
      |
      | This is all ok so long as you keep the ACK line high for an entire packet length.
  note: set until the first ack
  note: set during the second ack
  note: If the ack line goes low while there's still valid data on the output,
      | then we need to set the rd addr back one place and blank the next
      | output as invalid.
  note: Dualport ram incurrs delay
      | of one clock cycle
  din : Inport  Port=1  LatchInput=off
  we : Inport  Port=2  LatchInput=off
  commit : Inport  Port=3  LatchInput=off
  discard : Inport  Port=4  LatchInput=off
  ack : Inport  Port=5  LatchInput=off
  Constant5 : xbsIndex_r3/Constant  const=0  equ=P=C  arith_type=Boolean  n_bits=1  bin_pt=0  opselect=C  inp2=PCIN>>17  opr=+  inp1=P  carry=CIN  iostate=0  explicit_period=on  period=1  dbl_ovrd=off
  Delay : xbsIndex_r3/Delay  latency=1  reg_retiming=on  explicit_period=off  period=1  en=off  accept_only_valid=off  init_zero=on  dbl_ovrd=off  show_param=off
      settings: xl_area=[0, 0, 0, 0, 0, 0, 0]
  Delay15 : xbsIndex_r3/Delay  latency=1  reg_retiming=on  explicit_period=off  period=1  en=off  accept_only_valid=off  init_zero=on  dbl_ovrd=off  show_param=off
      settings: xl_area=[0, 0, 0, 0, 0, 0, 0]
  Dual Port RAM : xbsIndex_r3/Dual Port RAM  depth=2^depth_bits  initVector=0  write_mode_A=Read Before Write  write_mode_B=Read Before Write  latency=1  mem_collision=off  init_zero=on  explicit_period=off  period=1  dbl_ovrd=off  rst_a=off  init_a=0  rst_b=off  init_b=0  show_param=off  distributed_mem=off  use_rpm=off  gen_core=off
      settings: xl_area=[0, 0, 0, 0, 0, 0, 0]
  Gateway Out{1..12,22..25,39} (17 alike) : xbsIndex_r3/Gateway Out  output_type=Double  nbits=8  bin_pt=6  arith_type=Boolean  quantization=Truncate  overflow=Wrap  hdl_port=on  timing_constraint=None  locs_specified=off  LOCs={}  needs_fixed_name=off  show_param=off
      settings: xl_area=[0, 0, 0, 0, 0, 0, 0]
  Inverter{1,3..8} (7 alike) : xbsIndex_r3/Inverter  latency=0  explicit_period=off  period=1  en=off  dbl_ovrd=off  show_param=off
      settings: xl_area=[0, 0, 0, 0, 0, 0, 0]
  Inverter2 : xbsIndex_r3/Inverter  Orientation=up  latency=0  explicit_period=off  period=1  en=off  dbl_ovrd=off  show_param=off
      settings: xl_area=[0, 0, 0, 0, 0, 0, 0]
  Logical : xbsIndex_r3/Logical  logical_function=OR  inputs=2  precision=Full  arith_type=Unsigned  n_bits=8  bin_pt=2  align_bp=on  latency=0  explicit_period=off  period=1  en=off  dbl_ovrd=off  show_param=off
      settings: xl_area=[0, 0, 0, 0, 0, 0, 0]
  Logical1 : xbsIndex_r3/Logical  logical_function=AND  inputs=2  precision=Full  arith_type=Unsigned  n_bits=8  bin_pt=2  align_bp=on  latency=0  explicit_period=on  period=1  en=off  dbl_ovrd=off  show_param=off
      settings: xl_area=[0, 0, 0, 0, 0, 0, 0]
  Logical2 : xbsIndex_r3/Logical  logical_function=AND  inputs=3  precision=Full  arith_type=Unsigned  n_bits=8  bin_pt=2  align_bp=on  latency=0  explicit_period=on  period=1  en=off  dbl_ovrd=off  show_param=off
      settings: xl_area=[0, 0, 0, 0, 0, 0, 0]
  Logical{3..4,6,8..9} (5 alike) : xbsIndex_r3/Logical  logical_function=AND  inputs=2  precision=Full  arith_type=Unsigned  n_bits=8  bin_pt=2  align_bp=on  latency=0  explicit_period=off  period=1  en=off  dbl_ovrd=off  show_param=off
      settings: xl_area=[0, 0, 0, 0, 0, 0, 0]
  Logical5 : xbsIndex_r3/Logical  logical_function=XOR  inputs=2  precision=Full  arith_type=Unsigned  n_bits=8  bin_pt=2  align_bp=on  latency=0  explicit_period=off  period=1  en=off  dbl_ovrd=off  show_param=off
      settings: xl_area=[0, 0, 0, 0, 0, 0, 0]
  Logical7 : xbsIndex_r3/Logical  logical_function=OR  inputs=2  precision=Full  arith_type=Unsigned  n_bits=8  bin_pt=2  align_bp=on  latency=0  explicit_period=off  period=1  en=off  dbl_ovrd=off  show_param=off
      settings: xl_area=[0, 0, 0, 0, 0, 0, 0]
  Register : xbsIndex_r3/Register  init=0  reg_only_valid=off  explicit_period=on  period=1  rst=off  en=on  out_en=off  dbl_ovrd=off  show_param=off
      settings: xl_area=[0, 0, 0, 0, 0, 0, 0]
  Register1 : xbsIndex_r3/Register  init=0  reg_only_valid=off  explicit_period=on  period=1  rst=on  en=on  out_en=off  dbl_ovrd=off  show_param=off
      settings: xl_area=[0, 0, 0, 0, 0, 0, 0]
  Register2 : xbsIndex_r3/Register  init=0  reg_only_valid=off  explicit_period=on  period=1  rst=on  en=on  out_en=off  dbl_ovrd=off  show_param=off
      settings: xl_area=[0, 0, 0, 0, 0, 0, 0]
  Relational1 : xbsIndex_r3/Relational  mode=a=b  latency=0  explicit_period=on  period=1  en=off  dbl_ovrd=off  show_param=off
      settings: xl_area=[0, 0, 0, 0, 0, 0, 0]
  Relational2 : xbsIndex_r3/Relational  mode=a=b  latency=0  explicit_period=on  period=1  en=off  dbl_ovrd=off  show_param=off
      settings: xl_area=[0, 0, 0, 0, 0, 0, 0]
  Slice : xbsIndex_r3/Slice  mode=Two Bit Locations  nbits=1  bit1=-1  base1=MSB of Input  bit0=0  base0=LSB of Input  boolean_output=off  explicit_period=off  period=1  dbl_ovrd=off
  Slice1 : xbsIndex_r3/Slice  mode=Upper Bit Location + Width  nbits=1  bit1=0  base1=MSB of Input  bit0=0  base0=LSB of Input  boolean_output=on  explicit_period=off  period=1  dbl_ovrd=off
  Slice2 : xbsIndex_r3/Slice  mode=Two Bit Locations  nbits=1  bit1=-1  base1=MSB of Input  bit0=0  base0=LSB of Input  boolean_output=off  explicit_period=off  period=1  dbl_ovrd=off
  Slice3 : xbsIndex_r3/Slice  mode=Upper Bit Location + Width  nbits=1  bit1=0  base1=MSB of Input  bit0=0  base0=LSB of Input  boolean_output=on  explicit_period=off  period=1  dbl_ovrd=off
  ack_cnt : xbsIndex_r3/Counter  cnt_type=Free Running  n_bits=depth_bits + 1  bin_pt=0  arith_type=Unsigned  start_count=0  cnt_to=Inf  cnt_by_val=1  operation=Up  explicit_period=on  period=1  load_pin=off  rst=off  en=on  dbl_ovrd=off  show_param=off  use_rpm=on  gen_core=off
      settings: xl_area=[0, 0, 0, 0, 0, 0, 0]
  buf_debug : Scope  NumInputPorts=10
      settings: YMin=12000~0~9500~0~15500~-5~-5~-5~-5~-5  YMax=13300~1~10500~1~17250~5~5~5~5~5  SaveName=ScopeData13
  buf_debug2 : Scope  NumInputPorts=4
      settings: YMin=0~1~0~-1  YMax=1~1~1~1  SaveName=ScopeData15
  negedge : casper_library/Misc/negedge  Tag=Rising Edge Detector
  negedge2 : casper_library/Misc/negedge  Tag=Rising Edge Detector
  rd_cnt : xbsIndex_r3/Counter  cnt_type=Free Running  n_bits=depth_bits + 1  bin_pt=0  arith_type=Unsigned  start_count=0  cnt_to=Inf  cnt_by_val=1  operation=Up/Down  explicit_period=on  period=1  load_pin=off  rst=off  en=on  dbl_ovrd=off  show_param=off  use_rpm=on  gen_core=off
      settings: xl_area=[0, 0, 0, 0, 0, 0, 0]
  rd_wr_debug : Scope  NumInputPorts=3
      settings: YMin=12000~0~-5  YMax=13300~1~5  SaveName=ScopeData14
  set_cnt : Subsystem
  wr_cnt : xbsIndex_r3/Counter  cnt_type=Free Running  n_bits=depth_bits + 1  bin_pt=0  arith_type=Unsigned  start_count=0  cnt_to=Inf  cnt_by_val=1  operation=Up  explicit_period=on  period=1  load_pin=off  rst=off  en=on  dbl_ovrd=off  show_param=off  use_rpm=on  gen_core=off
      settings: xl_area=[0, 0, 0, 0, 0, 0, 0]
  dout : Outport
  valid : Outport  Port=2
  wr_ack : Outport  Port=3
  full : Outport  Port=4
  empty : Outport  Port=5
  wires:
  Relational2/1 -> Logical1/1
  Logical6/1 -> Inverter2/1, full/1
  Logical5/1 -> Logical6/1
  Relational1/1 -> Logical6/2
  Slice1/1 -> Logical5/2
  Slice3/1 -> Logical5/1
  Slice2/1 -> Relational1/1, Dual Port RAM/1
  Slice/1 -> Relational1/2, Dual Port RAM/4
  set_cnt/2(cnt) -> Slice3/1, Slice2/1, [wr_cnt]
  set_cnt/1(set_cnt) -> Relational2/1
  rd_cnt/1 -> [rd_cnt], Slice/1
  commit/1 -> [commit]
  Inverter2/1 -> Logical1/2, Logical3/2
  we/1 -> [we]
  discard/1 -> set_cnt/2(undo)
  Constant5/1 -> Dual Port RAM/6
  Dual Port RAM/2 -> dout/1, [dout]
  Logical1/1 -> [empty], Delay15/1
  Gateway Out24/1 -> buf_debug/1
  Gateway Out2/1 -> buf_debug/2
  Gateway Out39/1 -> buf_debug/3
  Gateway Out25/1 -> buf_debug/4
  Gateway Out1/1 -> buf_debug/5
  Gateway Out22/1 -> buf_debug/6
  Gateway Out23/1 -> buf_debug/7
  Gateway Out3/1 -> buf_debug/8
  Gateway Out4/1 -> buf_debug/9
  ack_cnt/1 -> Gateway Out3/1
  wr_cnt/1 -> Gateway Out4/1
  [empty] -> Inverter1/1
  [v_out] -> Gateway Out22/1
  ack/1 -> [ack_out], negedge2/1
  [ack_out] -> Logical4/1
  [ack_out] -> ack_cnt/1
  [ack_out] -> Gateway Out23/1
  Gateway Out6/1 -> rd_wr_debug/1
  Gateway Out5/1 -> rd_wr_debug/2
  Gateway Out7/1 -> rd_wr_debug/3
  [ack_out] -> Gateway Out7/1
  Gateway Out8/1 -> buf_debug/10
  [empty] -> Gateway Out8/1
  Inverter1/1 -> Logical4/2
  Logical2/1 -> valid/1, [v_out]
  [ack_negedge] -> Register1/1, Register1/3, Register2/2
  [ack_out] -> Register1/2
  Register1/1 -> Register2/1
  Gateway Out10/1 -> buf_debug2/1
  Gateway Out9/1 -> buf_debug2/2
  Gateway Out12/1 -> buf_debug2/3
  Gateway Out11/1 -> buf_debug2/4
  [ack_out] -> Gateway Out9/1
  [empty] -> Gateway Out10/1
  [v_out] -> Gateway Out12/1
  [ack_out] -> Register2/3
  [wr_ack] -> wr_cnt/1
  [wr_cnt] -> Gateway Out6/1
  [rd_cnt] -> Gateway Out5/1
  [wr_ack] -> Gateway Out39/1
  [commit] -> Gateway Out25/1
  [dout] -> Gateway Out1/1
  [we] -> Gateway Out2/1
  [din] -> Gateway Out24/1
  [commit] -> set_cnt/1(set)
  [wr_ack] -> Dual Port RAM/3
  [wr_ack] -> set_cnt/3(en)
  [we] -> Logical3/1
  Logical3/1 -> wr_ack/1, [wr_ack]
  [din] -> Dual Port RAM/2, Dual Port RAM/5
  din/1 -> [din]
  [rd_cnt] -> Slice1/1
  [rd_cnt] -> Relational2/2
  Register2/1 -> Gateway Out11/1, Inverter4/1
  negedge2/1 -> [ack_negedge]
  Inverter6/1 -> rd_cnt/1
  Logical7/1 -> rd_cnt/2
  Logical4/1 -> Logical7/2
  Logical8/1 -> Inverter6/1, Logical7/1
  [ack_negedge] -> Logical8/1
  [empty_out] -> Inverter7/1
  Inverter7/1 -> Logical8/2
  [ack_negedge] -> Logical9/1
  [empty_out] -> Inverter5/1
  Inverter5/1 -> Logical9/2
  Logical9/1 -> Delay/1
  Delay/1 -> Inverter8/1
  Inverter3/1 -> Register/1
  [empty] -> Inverter3/1
  Logical/1 -> Register/2
  [empty] -> negedge/1
  [ack_out] -> Logical/1
  negedge/1 -> Logical/2
  Inverter4/1 -> Logical2/3
  Inverter8/1 -> Logical2/1
  Register/1 -> Logical2/2
  Delay15/1 -> empty/1, [empty_out]
